simulink model "MPSK_model1"  (Simulink 7.6)
settings: Solver=FixedStepDiscrete  SolverMode=SingleTasking  StartTime=0.0  StopTime=1  FixedStep=1/100000  RelTol=1e-3  AbsTol=1e-6
PreLoadFcn:
  | fs=100000; Ts=1/fs; R=1000; T=1/R; fc=10000; M=8;
undefined symbols (not defined in the file): get
libraries: simulink x4, commsink2 x2, commfilt2 x2, commutil2 x1, simulink_extras x1, commrandsrc2 x1
settings Model: Creator=amoura  LastModifiedBy=Sílvio
settings DataIOCC: LimitDataPoints=off
settings OptimizationCC: BlockReduction=off  BooleanDataType=off  InitFltsAndDblsToZero=on
settings DebuggingCC: SaveWithParameterizedLinksMsg=none  SignalResolutionControl=TryResolveAllWithWarning  SolverPrmCheckMsg=none  MultiTaskDSMMsg=warning  MultiTaskCondExecSysMsg=none  StrictBusMsg=None
settings HardwareCC: TargetUnknown=on
settings RTWCC: TemplateMakefile=grt_unix.tmf  IncludeERTFirstTime=on
settings GRTTargetCC: TargetFcnLib=ansi_tfl_tmw.mat  ModelReferenceCompliant=off  MatFileLogging=off

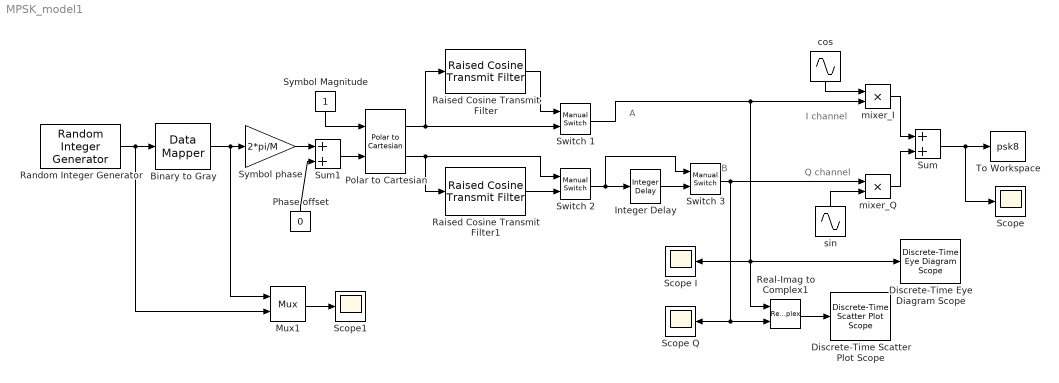
== system MPSK_model1 ==
  note: I channel
  note: Q channel
  note: A
  note: B
  Binary to Gray : commutil2/Data Mapper  SystemSampleTime=-1  MapMode=Binary to Gray  M=M  MapVec=[0 1 3 2 7 6 4 5]
  Discrete-Time Eye Diagram Scope : commsink2/Discrete-Time Eye Diagram Scope  Tag=EyeDiagram  SystemSampleTime=-1  sampPerSymb=100  offsetEye=0  symbPerTrace=2  numTraces=100  numNewFrames=4  LineStyles=-  LineColors=b  dupPoints=on  fading=on  render=on  AxisGrid=on  yMin=-1.44687388403113  yMax=1.37607599455112  inphaseLabel=In-phase Amplitude  quadratureLabel=Quadrature Amplitude  openScopeAtSimStart=on  dispDiagram=In-phase Only  FrameNumber=off  FigPos=get(0,'defaultfigureposition');  figTitle=Eye Diagram  block_type_=eye  numLinesMax=8
  Discrete-Time Scatter Plot Scope : commsink2/Discrete-Time Scatter Plot Scope  Tag=ScatterPlot  SystemSampleTime=-1  sampPerSymb=fs/R  offsetEye=0  numTraces=100  numNewFrames=100  LineMarkers=.  LineColors=b  fading=on  render=on  AxisGrid=on  xMin=-1.05  xMax=1.05  yMin=-1.05  yMax=1.05  inphaseLabel=In-phase Amplitude  quadratureLabel=Quadrature Amplitude  openScopeAtSimStart=on  FrameNumber=off  FigPos=get(0,'defaultfigureposition');  figTitle=Scatter Plot  numLinesMax=8  block_type_=scatter
  Integer Delay : simulink/Discrete/Integer Delay  NumDelays=12  vinit=0  samptime=-1
  Mux1 : Mux  Inputs=2
  Phase offset : Constant  Value=0  SampleTime=T
  Polar to Cartesian : simulink_extras/Transformations/Polar to Cartesian  SystemSampleTime=-1
  Raised Cosine Transmit Filter : commfilt2/Raised Cosine Transmit Filter  DialogController=dspDDGCreate  DialogControllerArgs=DataTag2  SystemSampleTime=-1  filtType=Normal  D=4  R=0.5  sampMode=Mute  saveAsFlag=0  N=100  framing=Allow multirate processing  checkGain=Normalized  filterGain=1  checkCoeff=off  variableName=rcTxFilt  launchFVT=off  roundingMode=Floor  overflowMode=off
  Raised Cosine Transmit Filter1 : commfilt2/Raised Cosine Transmit Filter  DialogController=dspDDGCreate  DialogControllerArgs=DataTag4  SystemSampleTime=-1  filtType=Normal  D=4  R=0.5  sampMode=Mute  saveAsFlag=0  N=100  framing=Allow multirate processing  checkGain=Normalized  filterGain=1  checkCoeff=off  variableName=rcTxFilt1  launchFVT=off  roundingMode=Floor  overflowMode=off
  Random Integer Generator : commrandsrc2/Random Integer Generator  SystemSampleTime=-1  mul=M  seed=randseed  Ts=T  frameBased=off  sampPerFrame=1  orient=off  outDataType=double
  Real-Imag to Complex1 : RealImagToComplex
  Scope : Scope
      settings: TickLabels=on  TimeRange=0.01  YMin=-2  YMax=2  DataFormat=Array
  Scope I : Scope
      settings: TickLabels=on  TimeRange=0.01  YMin=-2  YMax=2  DataFormat=Array
  Scope Q : Scope
      settings: TickLabels=on  TimeRange=0.01  YMin=-2  YMax=2  SaveName=ScopeData3  DataFormat=Array
  Scope1 : Scope
      settings: TickLabels=on  YMin=-1  YMax=8  DataFormat=Array
  Sum : Sum  SampleTime=Ts  SaturateOnIntegerOverflow=on  InputSameDT=on  OutDataTypeStr=Inherit: Same as first input
  Sum1 : Sum  SaturateOnIntegerOverflow=on  InputSameDT=on  OutDataTypeStr=Inherit: Same as first input
  Switch 1 : simulink/Signal Routing/Manual Switch  SystemSampleTime=-1  sw=1  action=0  varsize=off
  Switch 2 : simulink/Signal Routing/Manual Switch  SystemSampleTime=-1  sw=0  action=0  varsize=off
  Switch 3 : simulink/Signal Routing/Manual Switch  SystemSampleTime=-1  sw=1  action=0  varsize=off
  Symbol Magnitude : Constant  SampleTime=T
  Symbol phase : Gain  Gain=2*pi/M  SaturateOnIntegerOverflow=on  OutDataTypeStr=Inherit: Same as input  ParamDataTypeStr=Inherit: Same as input
  To Workspace : ToWorkspace  VariableName=psk8  SampleTime=Ts  SaveFormat=Array
  cos : Sin  Frequency=2*pi*fc  Phase=pi/2  SampleTime=0
  mixer_I : Product  SampleTime=Ts  SaturateOnIntegerOverflow=on  RndMeth=Zero  InputSameDT=on  OutDataTypeStr=Inherit: Same as first input
  mixer_Q : Product  SampleTime=Ts  SaturateOnIntegerOverflow=on  RndMeth=Zero  InputSameDT=on  OutDataTypeStr=Inherit: Same as first input
  sin : Sin  Frequency=2*pi*fc  SampleTime=0
  wires:
  Mux1/1 -> Scope1/1
  Binary to Gray/1 -> Mux1/1, Symbol phase/1
  Random Integer Generator/1 -> Mux1/2, Binary to Gray/1
  Symbol Magnitude/1 -> Polar to Cartesian/1
  mixer_I/1 -> Sum/1
  mixer_Q/1 -> Sum/2
  sin/1 -> mixer_Q/2
  cos/1 -> mixer_I/1
  Sum/1 -> To Workspace/1, Scope/1
  Switch 1/1 -> mixer_I/2, Real-Imag to Complex1/1, Discrete-Time Eye Diagram Scope/1, Scope I/1
  Switch 2/1 -> Switch 3/1, Integer Delay/1
  Polar to Cartesian/1 -> Switch 1/2, Raised Cosine Transmit Filter/1
  Raised Cosine Transmit Filter/1 -> Switch 1/1
  Polar to Cartesian/2 -> Switch 2/1, Raised Cosine Transmit Filter1/1
  Raised Cosine Transmit Filter1/1 -> Switch 2/2
  Integer Delay/1 -> Switch 3/2
  Switch 3/1 -> mixer_Q/1, Real-Imag to Complex1/2, Scope Q/1
  Symbol phase/1 -> Sum1/1
  Sum1/1 -> Polar to Cartesian/2
  Phase offset/1 -> Sum1/2
  Real-Imag to Complex1/1 -> Discrete-Time Scatter Plot Scope/1
